simulink subsystem "mfc_F_est_cont_coupled"  (R2026a)
settings: Solver=VariableStepAuto
settings Model: Creator=devinbellll  LastModifiedBy=devinbellll

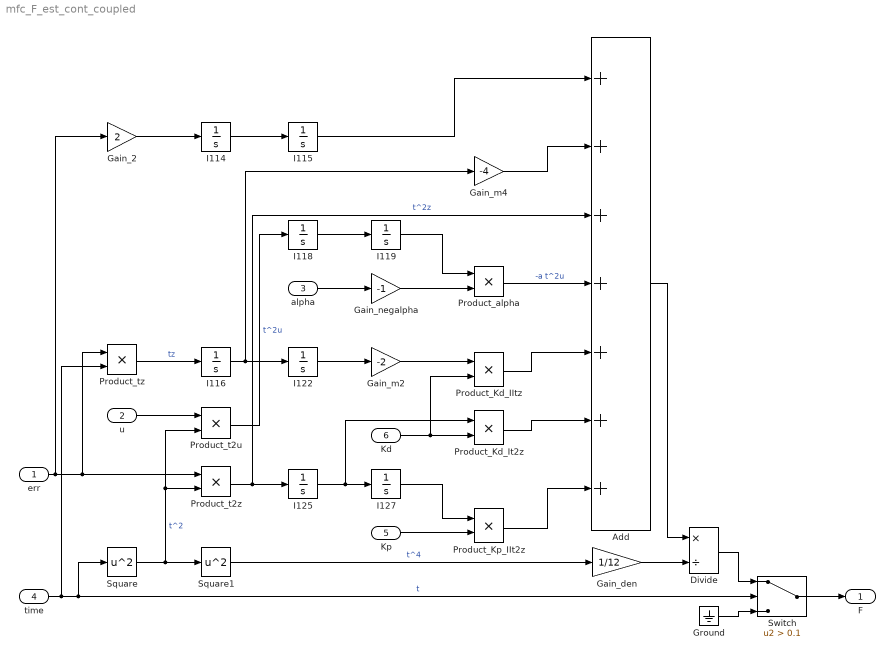
== system mfc_F_est_cont_coupled ==
  err : Inport
  u : Inport  Port=2
  alpha : Inport  Port=3
  time : Inport  Port=4
  Kp : Inport  Port=5
  Kd : Inport  Port=6
  Add : Sum  Inputs=+++++++
  Divide : Product  Inputs=*/
  Gain_2 : Gain  Gain=2
  Gain_den : Gain  Gain=1/12
  Gain_m2 : Gain  Gain=-2
  Gain_m4 : Gain  Gain=-4
  Gain_negalpha : Gain  Gain=-1
  Ground : Ground
  I{114..116,118..119,122,125,127} (8 alike) : Integrator
  Product_Kd_IItz : Product
  Product_Kd_It2z : Product
  Product_Kp_IIt2z : Product
  Product_alpha : Product
  Product_t2u : Product
  Product_t2z : Product
  Product_tz : Product
  Square : Math  Operator=square
  Square1 : Math  Operator=square
  Switch : Switch  Criteria=u2 > Threshold  Threshold=0.1  SaturateOnIntegerOverflow=off  InputSameDT=off
  F : Outport
  wires:
  Switch/1 -> F/1
  Divide/1 -> Switch/1
  Add/1 -> Divide/1
  Product_Kp_IIt2z/1 -> Add/7
  Product_Kd_IItz/1 -> Add/5
  Product_alpha/1 -> Add/4  "-a t^2u"
  Kp/1 -> Product_Kp_IIt2z/2
  Gain_m2/1 -> Product_Kd_IItz/1
  Kd/1 -> Product_Kd_It2z/2, Product_Kd_IItz/2
  Gain_m4/1 -> Add/2
  I119/1 -> Product_alpha/1
  I125/1 -> I127/1, Product_Kd_It2z/1
  Gain_negalpha/1 -> Product_alpha/2
  Product_tz/1 -> I116/1  "tz"
  Product_t2z/1 -> I125/1, Add/3  "t^2z"
  Square1/1 -> Gain_den/1  "t^4"
  I122/1 -> Gain_m2/1
  err/1 -> Product_t2z/1, Product_tz/1, Gain_2/1
  I116/1 -> I122/1, Gain_m4/1
  I114/1 -> I115/1
  I115/1 -> Add/1
  Product_Kd_It2z/1 -> Add/6
  u/1 -> Product_t2u/1
  Ground/1 -> Switch/3
  Product_t2u/1 -> I118/1  "t^2u"
  Gain_2/1 -> I114/1
  I118/1 -> I119/1
  time/1 -> Square/1, Switch/2, Product_tz/2  "t"
  I127/1 -> Product_Kp_IIt2z/1
  Gain_den/1 -> Divide/2
  alpha/1 -> Gain_negalpha/1
  Square/1 -> Product_t2z/2, Product_t2u/2, Square1/1  "t^2"
